simulink model "e_Aerodynamics_added"  (R2025b)
settings: Solver=ode23tb  StartTime=0.0  StopTime=20  MaxStep=0.001  RelTol=1e-3
model workspace (MAT data in the model file):
  init_r = 0
  init_vx = 0
  init_vy = 0
values from neighbouring files (symbols this model uses):
  Par =     [0_Load_data.mat]
  TireData =     [0_Load_data.mat]
libraries: simulink x3
(part 1 of 2)
settings Model: PauseTimes=0  PacingRate=0.001000  Creator=rajde  LastModifiedBy=vishal bhujbal
settings DataIOCC: SaveOutput=off  SaveTime=off
settings DebuggingCC: UnderSpecifiedDimensionMsg=warning

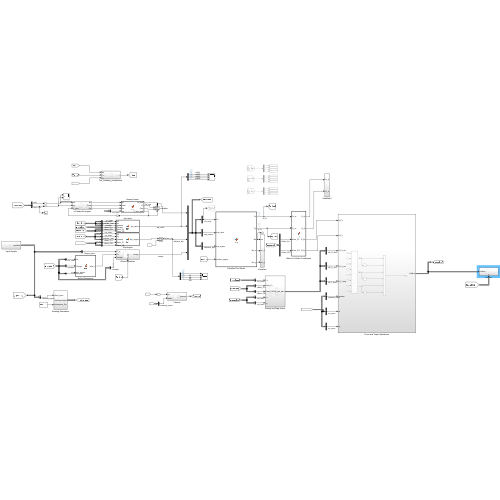
[thumbnail: Simulink's stored preview of the top-level diagram]
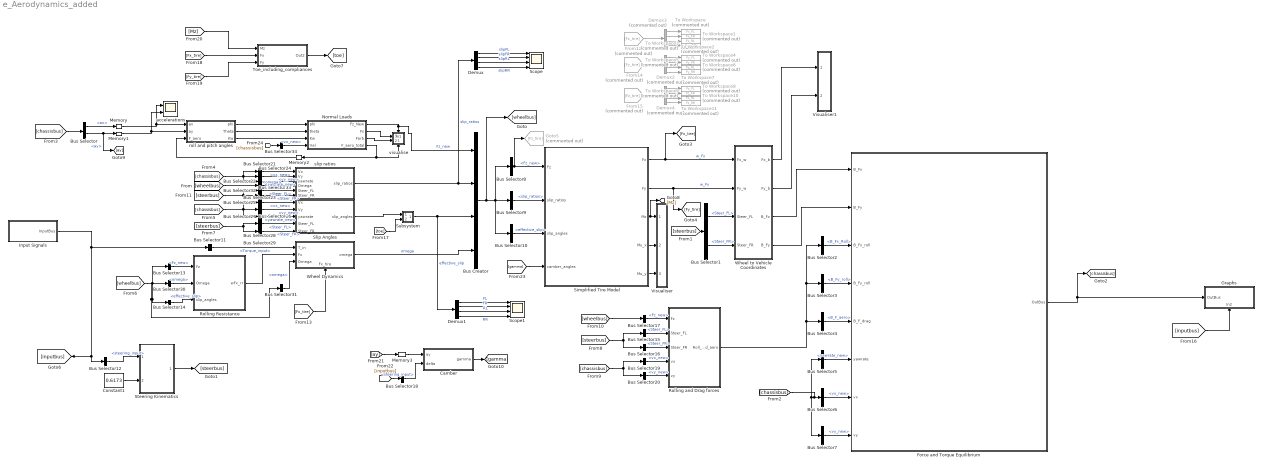
== system e_Aerodynamics_added ==
  Bus Creator : BusCreator  Inputs=4
  Bus Selector : BusSelector  OutputSignals=ax,ay
  Bus Selector1 : BusSelector  OutputSignals=Steer_FL,Steer_FR
  Bus Selector10 : BusSelector  OutputSignals=effective_slip
  Bus Selector11 : BusSelector  OutputSignals=Torque_input
  Bus Selector12 : BusSelector  OutputSignals=steering_input
  Bus Selector13 : BusSelector  OutputSignals=Fz_new
  Bus Selector14 : BusSelector  OutputSignals=effective_slip
  Bus Selector15 : BusSelector  OutputSignals=Steer_FL
  Bus Selector16 : BusSelector  OutputSignals=Steer_FR
  Bus Selector17 : BusSelector  OutputSignals=Fz_new
  Bus Selector18 : BusSelector  OutputSignals=steering_input
  Bus Selector{6,19,21,25,34} (5 alike) : BusSelector  OutputSignals=vx_new
  Bus Selector2 : BusSelector  OutputSignals=B_Fx_Roll
  Bus Selector{7,20,24,26} (4 alike) : BusSelector  OutputSignals=vy_new
  Bus Selector22 : BusSelector  OutputSignals=yawrate_new
  Bus Selector23 : BusSelector  OutputSignals=omega
  Bus Selector27 : BusSelector  OutputSignals=yawrate_new
  Bus Selector28 : BusSelector  OutputSignals=Steer_FL
  Bus Selector29 : BusSelector  OutputSignals=Steer_FR
  Bus Selector3 : BusSelector  OutputSignals=B_Fy_roll
  Bus Selector30 : BusSelector  OutputSignals=omega
  Bus Selector31 : BusSelector  OutputSignals=omega
  Bus Selector32 : BusSelector  OutputSignals=Steer_FL
  Bus Selector33 : BusSelector  OutputSignals=Steer_FR
  Bus Selector4 : BusSelector  OutputSignals=B_F_aero
  Bus Selector5 : BusSelector  OutputSignals=yawrate_new
  Bus Selector8 : BusSelector  OutputSignals=Fz_new
  Bus Selector9 : BusSelector  OutputSignals=slip_ratios
  Camber : Subsystem
  Constant1 : Constant  Value=0.6173
  Demux : Demux
  Demux1 : Demux
  Demux2 : Demux  Commented=on
  Demux3 : Demux  Commented=on
  Demux4 : Demux  Commented=on
  Force and Torque Equilibrium : Subsystem
  From12 : From  Commented=on  GotoTag=Fx_tire
  From14 : From  Commented=on  GotoTag=Fy_tire
  From15 : From  Commented=on  GotoTag=Fz_tire
  Goto5 : Goto  Commented=on  GotoTag=Fz_tire
  Graphs : Subsystem
      settings: PortSchema="{\"entries\":[{\"content\":{\"sides\":[{\"content\":{\"connectorIds\":[\"In1\"]},\"type\":\"ConnectorPlacement.EquallySpacedRectSide\",\"uuid\":\"0d7f1a6c-503e-4c9f-90e9-70f717dd7dfc\"},{\"content\":{\"side\":\"RIGHT\"},\"type\":\"ConnectorPlacement.EquallySpacedRectSide\",\"uuid\":\"62097468-b066-4e29-8f99-7427d14bee77\"},{\"content\":{\"side\":\"TOP\"},\"type\":\"ConnectorPlacement.EquallySpacedRectSide\",\"uuid\":\"2a3f381e-a201-4804-99b7-77b73504b102\"},{\"content\":{\"connectorIds\":[\"In2\"],\"side\":\"BOTTOM\"},\"type\":\"ConnectorPlacement.EquallySpacedRectSide\",\"uuid\":\"dae5de0a-879c-4844-a347-7056417d054f\"}]},\"type\":\"ConnectorPlacement.EquallySpacedConnector\",\"uuid\":\"aa2835d0-6748-4566-adf9-84e8214dd5a8\"}],\"packageUris\":[\"http://schema.mathworks.com/mf0/Connector/R2020b\"],\"version\":\"1.0\"}"
  Input Signals : Subsystem
  Memory : Memory  InheritSampleTime=on
  Memory1 : Memory  InheritSampleTime=on
  Memory2 : Memory  InheritSampleTime=on
  Memory3 : Memory
  Normal Loads : MATLAB Function  TreatAsAtomicUnit=on
  Rolling Resistance : MATLAB Function  TreatAsAtomicUnit=on
  Rolling and Drag forces : Subsystem
  Scope : Scope  NumInputPorts=4
      settings: ActiveDisplayYMinimum=-0.00902343797023162  ActiveDisplayYMaximum=0.049451714787091476  DataLoggingVariableName=ScopeData3
  Scope1 : Scope  NumInputPorts=4
      settings: ActiveDisplayYMinimum=-0.4830772017663526  ActiveDisplayYMaximum=0.53547210256097  DataLoggingVariableName=ScopeData4
  Simplified Tire Model : MATLAB Function  TreatAsAtomicUnit=on
  Slip Angles : MATLAB Function  TreatAsAtomicUnit=on
  Steering Kinematics : Subsystem
  Subsystem : Subsystem
  To Workspace : ToWorkspace  Commented=on  VariableName=Fx_FL  SaveFormat=Timeseries  SampleTime=-1
  To Workspace1 : ToWorkspace  Commented=on  VariableName=Fx_FR  SaveFormat=Timeseries  SampleTime=-1
  To Workspace10 : ToWorkspace  Commented=on  VariableName=Fz_RL  SaveFormat=Timeseries  SampleTime=-1
  To Workspace11 : ToWorkspace  Commented=on  VariableName=Fz_RR  SaveFormat=Timeseries  SampleTime=-1
  To Workspace2 : ToWorkspace  Commented=on  VariableName=Fx_RL  SaveFormat=Timeseries  SampleTime=-1
  To Workspace3 : ToWorkspace  Commented=on  VariableName=Fx_RR  SaveFormat=Timeseries  SampleTime=-1
  To Workspace4 : ToWorkspace  Commented=on  VariableName=Fy_FL  SaveFormat=Timeseries  SampleTime=-1
  To Workspace5 : ToWorkspace  Commented=on  VariableName=Fy_FR  SaveFormat=Timeseries  SampleTime=-1
  To Workspace6 : ToWorkspace  Commented=on  VariableName=Fy_RL  SaveFormat=Timeseries  SampleTime=-1
  To Workspace7 : ToWorkspace  Commented=on  VariableName=Fy_RR  SaveFormat=Timeseries  SampleTime=-1
  To Workspace8 : ToWorkspace  Commented=on  VariableName=Fz_FL  SaveFormat=Timeseries  SampleTime=-1
  To Workspace9 : ToWorkspace  Commented=on  VariableName=Fz_FR  SaveFormat=Timeseries  SampleTime=-1
  Toe_including_compliances : Subsystem
  Visualiser : Subsystem
  Visualiser1 : Subsystem
  Wheel Dynamics : Subsystem
      settings: PortSchema="{\"entries\":[{\"content\":{\"sides\":[{\"content\":{\"connectorIds\":[\"In1\",\"In2\",\"In3\"]},\"type\":\"ConnectorPlacement.EquallySpacedRectSide\",\"uuid\":\"f2e918e6-c6f6-4ec9-89f3-e2543a6374fd\"},{\"content\":{\"connectorIds\":[\"Out1\"],\"side\":\"RIGHT\"},\"type\":\"ConnectorPlacement.EquallySpacedRectSide\",\"uuid\":\"be700f5f-5cf3-4eec-a6f7-872bb7cd40f6\"},{\"content\":{\"side\":\"TOP\"},\"type\":\"ConnectorPlacement.EquallySpacedRectSide\",\"uuid\":\"c4f49273-9888-4d11-a98e-35dc6f585916\"},{\"content\":{\"connectorIds\":[\"In4\"],\"side\":\"BOTTOM\"},\"type\":\"ConnectorPlacement.EquallySpacedRectSide\",\"uuid\":\"8d2e7982-4362-4abb-b8fe-c155beeed1bc\"}]},\"type\":\"ConnectorPlacement.EquallySpacedConnector\",\"uuid\":\"4d6dafa1-905e-4e38-a48b-73a98e690073\"}],\"packageUris\":[\"http://schema.mathworks.com/mf0/Connector/R2020b\"],\"version\":\"1.0\"}"
  Wheel to Vehicle Coordinates : MATLAB Function  TreatAsAtomicUnit=on
  accelerations : Scope  NumInputPorts=2
      settings: ActiveDisplayYMinimum=-9.8753419220215122  ActiveDisplayYMaximum=20.918858613729107  DataLoggingVariableName=ScopeData12
  roll and pitch angles : Subsystem
  slip ratios : MATLAB Function  TreatAsAtomicUnit=on
  visualise : Subsystem
      settings: PortSchema="{\"entries\":[{\"content\":{\"sides\":[{\"content\":{\"connectorIds\":[\"In1\"]},\"type\":\"ConnectorPlacement.EquallySpacedRectSide\",\"uuid\":\"8366d134-d050-42cc-b256-e51a937b8428\"},{\"content\":{\"connectorIds\":[\"In4\"],\"side\":\"RIGHT\"},\"type\":\"ConnectorPlacement.EquallySpacedRectSide\",\"uuid\":\"98870c85-a760-468e-85de-3959de32b175\"},{\"content\":{\"connectorIds\":[\"In2\",\"In3\"],\"side\":\"TOP\"},\"type\":\"ConnectorPlacement.EquallySpacedRectSide\",\"uuid\":\"b49e1108-902f-401f-be37-4fefd9726c90\"}]},\"type\":\"ConnectorPlacement.EquallySpacedConnector\",\"uuid\":\"4200efe4-5812-4945-a73f-d6022d642a21\"}],\"packageUris\":[\"http://schema.mathworks.com/mf0/Connector/R2020b\"],\"version\":\"1.0\"}"
  wires:
  Simplified Tire Model/3(Mz) -> [Mz], Visualiser/1(mz)
  Simplified Tire Model/4(Mu_x) -> Visualiser/2(mu_x)
  Simplified Tire Model/5(Mu_y) -> Visualiser/3(mu_y)
  Simplified Tire Model/2(Fy) -> Wheel to Vehicle Coordinates/2(Fy_w), [Fy_tire]  "w_Fy"
  Simplified Tire Model/1(Fx) -> Wheel to Vehicle Coordinates/1(Fx_w), [Fx_tire]  "w_Fx"
  Wheel to Vehicle Coordinates/2(Fy_b) -> Visualiser1/2(Fy_b)
  Wheel to Vehicle Coordinates/1(Fx_b) -> Visualiser1/1(Fx_b)
  Wheel to Vehicle Coordinates/3(B_Fx) -> Force and Torque Equilibrium/1(B_Fx)
  Wheel to Vehicle Coordinates/4(B_Fy) -> Force and Torque Equilibrium/2(B_Fy)
  slip ratios/1(slip_ratios) -> Demux/1, Bus Creator/2  "slip_ratios"
  Wheel Dynamics/1(omega) -> Bus Creator/4  "omega"
  Bus Selector/1 -> Memory/1  "<ax>"
  Rolling Resistance/1(wFx_rr) -> Wheel Dynamics/2(Fx)
  Bus Selector1/1 -> Wheel to Vehicle Coordinates/3(Steer_FL)  "<Steer_FL>"
  Bus Selector1/2 -> Wheel to Vehicle Coordinates/4(Steer_FR)  "<Steer_FR>"
  Rolling and Drag forces/1(Roll_and_aero) -> Bus Selector2/1, Bus Selector3/1, Bus Selector4/1
  Bus Selector2/1 -> Force and Torque Equilibrium/3(B_Fx_roll)  "<B_Fx_Roll>"
  Bus Selector3/1 -> Force and Torque Equilibrium/4(B_Fy_roll)  "<B_Fy_roll>"
  Bus Selector4/1 -> Force and Torque Equilibrium/5(B_F_drag)  "<B_F_aero>"
  Bus Selector5/1 -> Force and Torque Equilibrium/6(yawrate)  "<yawrate_new>"
  Force and Torque Equilibrium/1(OutBus) -> [chassisbus], Graphs/1(OutBus)
  Bus Selector7/1 -> Force and Torque Equilibrium/8(vy)  "<vy_new>"
  Bus Selector6/1 -> Force and Torque Equilibrium/7(vx)  "<vx_new>"
  Bus Selector8/1 -> Goto5/1, Simplified Tire Model/1(Fz)  "<Fz_new>"
  Bus Selector10/1 -> Simplified Tire Model/3(slip_angles)  "<effective_slip>"
  Bus Selector9/1 -> Simplified Tire Model/2(slip_ratios)  "<slip_ratios>"
  Bus Creator/1 -> [wheelbus], Bus Selector10/1, Bus Selector8/1, Bus Selector9/1
  Bus Selector12/1 -> Steering Kinematics/1(Steer_Input)  "<steering_input>"
  Bus Selector11/1 -> Wheel Dynamics/1(T_in)  "<Torque_input>"
  Input Signals/1(InputBus) -> Bus Selector12/1, [inputbus], Bus Selector11/1
  Bus Selector14/1 -> Rolling Resistance/3(slip_angles)  "<effective_slip>"
  Bus Selector15/1 -> Rolling and Drag forces/2(Steer_FL)  "<Steer_FL>"
  Bus Selector16/1 -> Rolling and Drag forces/3(Steer_FR)  "<Steer_FR>"
  Constant1/1 -> Steering Kinematics/2(Ackermann_Pct)
  Bus Selector17/1 -> Rolling and Drag forces/1(Fz)  "<Fz_new>"
  Bus Selector19/1 -> Rolling and Drag forces/4(vx)  "<vx_new>"
  Bus Selector20/1 -> Rolling and Drag forces/5(vy)  "<vy_new>"
  Bus Selector21/1 -> slip ratios/1(Vx)  "<vx_new>"
  Bus Selector22/1 -> slip ratios/3(yawrate)  "<yawrate_new>"
  Bus Selector23/1 -> slip ratios/4(Omega)  "<omega>"
  Bus Selector25/1 -> Slip Angles/1(Vx)  "<vx_new>"
  Bus Selector26/1 -> Slip Angles/2(Vy)  "<vy_new>"
  Bus Selector27/1 -> Slip Angles/3(yawrate)  "<yawrate_new>"
  Bus Selector28/1 -> Slip Angles/4(Steer_FL)  "<Steer_FL>"
  Bus Selector29/1 -> Slip Angles/5(Steer_FR)  "<Steer_FR>"
  Steering Kinematics/1(Steering Angles) -> [steerbus]
  [steerbus] -> Bus Selector1/1
  [chassisbus] -> Bus Selector5/1, Bus Selector7/1, Bus Selector6/1
  [chassisbus] -> Bus Selector/1
  Bus Selector/2 -> Memory1/1, [ay]  "<ay>"
  [wheelbus] -> Bus Selector23/1
  [chassisbus] -> Bus Selector22/1, Bus Selector24/1, Bus Selector21/1
  [chassisbus] -> Bus Selector27/1, Bus Selector26/1, Bus Selector25/1
  [steerbus] -> Bus Selector29/1, Bus Selector28/1
  [wheelbus] -> Bus Selector13/1, Bus Selector30/1, Bus Selector14/1, Bus Selector31/1
  Bus Selector30/1 -> Rolling Resistance/2(Omega)  "<omega>"
  Bus Selector31/1 -> Wheel Dynamics/3(Omega)  "<omega>"
  [steerbus] -> Bus Selector16/1, Bus Selector15/1
  [chassisbus] -> Bus Selector20/1, Bus Selector19/1
  [wheelbus] -> Bus Selector17/1
  Demux/1 -> Scope/1  "slipFL"
  Demux/3 -> Scope/3  "slipRL"
  Demux/4 -> Scope/4  "slipRR"
  Demux/2 -> Scope/2  "slipFR"
  Demux1/1 -> Scope1/1  "FL"
  Demux1/2 -> Scope1/2  "FR"
  Demux1/4 -> Scope1/4  "RR"
  Demux1/3 -> Scope1/3  "RL"
  Bus Selector24/1 -> slip ratios/2(Vy)  "<vy_new>"
  Bus Selector33/1 -> slip ratios/6(Steer_FR)  "<Steer_FR>"
  [steerbus] -> Bus Selector32/1, Bus Selector33/1
  Bus Selector32/1 -> slip ratios/5(Steer_FL)  "<Steer_FL>"
  [Fx_tire] -> Wheel Dynamics/4(Fx_tire)
  Bus Selector13/1 -> Rolling Resistance/1(Fz)  "<Fz_new>"
  Demux2/2 -> To Workspace5/1
  Demux2/3 -> To Workspace6/1
  Demux3/3 -> To Workspace2/1
  Demux3/4 -> To Workspace3/1
  From12/1 -> Demux3/1
  From14/1 -> Demux2/1
  Demux3/2 -> To Workspace1/1
  Demux2/4 -> To Workspace7/1
  Demux3/1 -> To Workspace/1
  Demux2/1 -> To Workspace4/1
  Demux4/1 -> To Workspace8/1
  Demux4/4 -> To Workspace11/1
  Demux4/2 -> To Workspace9/1
  Demux4/3 -> To Workspace10/1
  From15/1 -> Demux4/1
  [inputbus] -> Graphs/2(In2)
  Slip Angles/1(slip_angles) -> Subsystem/1(slip_angles)
  [toe] -> Subsystem/2(toe)
  Subsystem/1(Out1) -> Demux1/1, Bus Creator/3  "effective_slip"
  [Mz] -> Toe_including_compliances/1(Mz)
  [Fx_tire] -> Toe_including_compliances/2(Fx)
  [Fy_tire] -> Toe_including_compliances/3(Fy)
  Toe_including_compliances/1(Out2) -> [toe]
  [ay] -> Memory3/1
  [inputbus] -> Bus Selector18/1
  Bus Selector18/1 -> Camber/2(delta)  "<steering_input>"
  Camber/1(gamma) -> [gamma]
  [gamma] -> Simplified Tire Model/4(camber_angles)
  roll and pitch angles/1(phi) -> Normal Loads/1(phi)
  roll and pitch angles/2(Theta) -> Normal Loads/2(theta)
  roll and pitch angles/3(Kw) -> Normal Loads/3(Kw)
  Normal Loads/1(Fz_New) -> Bus Creator/1, visualise/4(In1)  "Fz_new"
  Normal Loads/2(Fs) -> visualise/3(Fs)
  Normal Loads/3(Farb) -> visualise/2(Farb)
  Memory/1 -> accelerations/1, roll and pitch angles/1(ax)
  Memory1/1 -> roll and pitch angles/2(ay), accelerations/2
  Memory3/1 -> Camber/1(ay)
  Normal Loads/4(F_aero_total) -> visualise/1(F_aero_total), Memory2/1
  Memory2/1 -> roll and pitch angles/3(F_aero)
  [chassisbus] -> Bus Selector34/1
  Bus Selector34/1 -> Normal Loads/4(Vel)  "<vx_new>"

== system e_Aerodynamics_added/Camber ==
  ay : Inport
  delta : Inport  Port=2
  MATLAB Function : MATLAB Function  TreatAsAtomicUnit=on
  Mux : Mux
  gamma : Outport
  wires:
  MATLAB Function/1(gamma_FR) -> Mux/1
  MATLAB Function/2(gamma_FL) -> Mux/2
  MATLAB Function/3(gamma_RL) -> Mux/3
  MATLAB Function/4(gamma_RR) -> Mux/4
  Mux/1 -> gamma/1
  ay/1 -> MATLAB Function/1(ay)
  delta/1 -> MATLAB Function/2(delta)

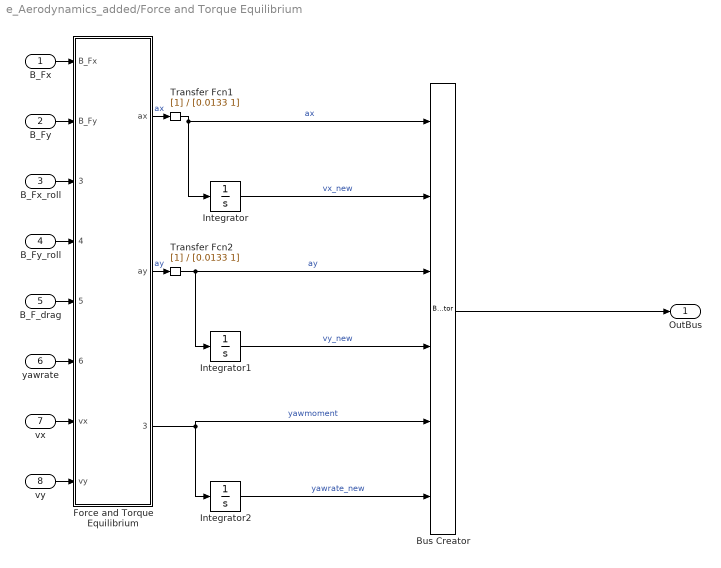
== system e_Aerodynamics_added/Force and Torque Equilibrium ==
  B_Fx : Inport
  B_Fy : Inport  Port=2
  B_Fx_roll : Inport  Port=3
  B_Fy_roll : Inport  Port=4
  B_F_drag : Inport  Port=5
  yawrate : Inport  Port=6
  vx : Inport  Port=7
  vy : Inport  Port=8
  Bus Creator : BusCreator  Inputs=6
  Force and Torque Equilibrium : MATLAB Function  TreatAsAtomicUnit=on
  Integrator : Integrator  LimitOutput=on  UpperSaturationLimit=1e6  LowerSaturationLimit=0
  Integrator1 : Integrator  LimitOutput=on  UpperSaturationLimit=1e6
  Integrator2 : Integrator  LimitOutput=on  UpperSaturationLimit=1e6
  Transfer Fcn1 : TransferFcn  Denominator=[0.0133 1]
  Transfer Fcn2 : TransferFcn  Denominator=[0.0133 1]
  OutBus : Outport
  wires:
  vy/1 -> Force and Torque Equilibrium/8(vy)
  B_Fx/1 -> Force and Torque Equilibrium/1(B_Fx)
  B_Fx_roll/1 -> Force and Torque Equilibrium/3(B_Fx_roll)
  B_F_drag/1 -> Force and Torque Equilibrium/5(B_F_drag)
  B_Fy/1 -> Force and Torque Equilibrium/2(B_Fy)
  B_Fy_roll/1 -> Force and Torque Equilibrium/4(B_Fy_roll)
  vx/1 -> Force and Torque Equilibrium/7(vx)
  Force and Torque Equilibrium/2(ay) -> Transfer Fcn2/1  "ay"
  Force and Torque Equilibrium/1(ax) -> Transfer Fcn1/1  "ax"
  Force and Torque Equilibrium/3(yawmoment) -> Integrator2/1, Bus Creator/5  "yawmoment"
  Integrator/1 -> Bus Creator/2  "vx_new"
  Integrator1/1 -> Bus Creator/4  "vy_new"
  Integrator2/1 -> Bus Creator/6  "yawrate_new"
  Bus Creator/1 -> OutBus/1
  yawrate/1 -> Force and Torque Equilibrium/6(yawrate)
  Transfer Fcn1/1 -> Integrator/1, Bus Creator/1  "ax"
  Transfer Fcn2/1 -> Integrator1/1, Bus Creator/3  "ay"

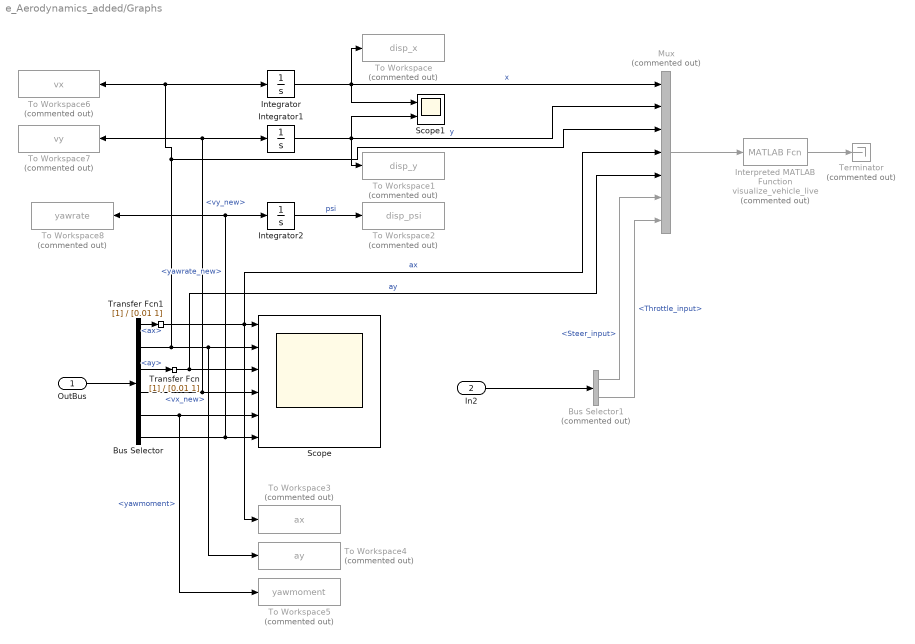
== system e_Aerodynamics_added/Graphs ==
  OutBus : Inport
  In2 : Inport  Port=2
  Bus Selector : BusSelector  OutputSignals=ax,vx_new,ay,vy_new,yawmoment,yawrate_new
  Bus Selector1 : BusSelector  Commented=on  OutputSignals=Steer_input,Throttle_input
  Integrator : Integrator
  Integrator1 : Integrator
  Integrator2 : Integrator
  Interpreted MATLAB Function : MATLABFcn  Commented=on  MATLABFcn=visualize_vehicle_live
  Mux : Mux  Commented=on  Inputs=7
  Scope : Scope  NumInputPorts=6
      settings: ActiveDisplayYMinimum=-1.8391798427639636  ActiveDisplayYMaximum=12.998606897592927  DataLoggingVariableName=ScopeData2
  Scope1 : Scope  NumInputPorts=2
      settings: ActiveDisplayYMinimum=-673.27901203322881  ActiveDisplayYMaximum=6059.5111082990607  DataLoggingVariableName=ScopeData7
  Terminator : Terminator  Commented=on
  To Workspace : ToWorkspace  Commented=on  VariableName=disp_x  SaveFormat=Timeseries  SampleTime=-1
  To Workspace1 : ToWorkspace  Commented=on  VariableName=disp_y  SaveFormat=Timeseries  SampleTime=-1
  To Workspace2 : ToWorkspace  Commented=on  VariableName=disp_psi  SaveFormat=Timeseries  SampleTime=-1
  To Workspace3 : ToWorkspace  Commented=on  VariableName=ax  SaveFormat=Timeseries  SampleTime=-1
  To Workspace4 : ToWorkspace  Commented=on  VariableName=ay  SaveFormat=Timeseries  SampleTime=-1
  To Workspace5 : ToWorkspace  Commented=on  VariableName=yawmoment  SaveFormat=Timeseries  SampleTime=-1
  To Workspace6 : ToWorkspace  Commented=on  VariableName=vx  SaveFormat=Timeseries  SampleTime=-1
  To Workspace7 : ToWorkspace  Commented=on  VariableName=vy  SaveFormat=Timeseries  SampleTime=-1
  To Workspace8 : ToWorkspace  Commented=on  VariableName=yawrate  SaveFormat=Timeseries  SampleTime=-1
  Transfer Fcn : TransferFcn  Denominator=[0.01 1]
  Transfer Fcn1 : TransferFcn  Denominator=[0.01 1]
  wires:
  OutBus/1 -> Bus Selector/1
  Bus Selector/1 -> Transfer Fcn1/1  "<ax>"
  Bus Selector/2 -> To Workspace6/1, Integrator/1, Mux/3, To Workspace4/1, Scope/2  "<vx_new>"
  Bus Selector/3 -> Transfer Fcn/1  "<ay>"
  Bus Selector/4 -> To Workspace7/1, Integrator1/1, Scope/4  "<vy_new>"
  Bus Selector/5 -> To Workspace5/1, Scope/5  "<yawmoment>"
  Bus Selector/6 -> To Workspace8/1, Integrator2/1, Scope/6  "<yawrate_new>"
  Integrator/1 -> Scope1/1, Mux/1, To Workspace/1  "x"
  Integrator1/1 -> Scope1/2, Mux/2, To Workspace1/1  "y"
  Integrator2/1 -> To Workspace2/1  "psi"
  Mux/1 -> Interpreted MATLAB Function/1
  Interpreted MATLAB Function/1 -> Terminator/1
  In2/1 -> Bus Selector1/1
  Bus Selector1/1 -> Mux/6  "<Steer_input>"
  Bus Selector1/2 -> Mux/7  "<Throttle_input>"
  Transfer Fcn/1 -> Mux/5, Scope/3  "ay"
  Transfer Fcn1/1 -> To Workspace3/1, Scope/1, Mux/4  "ax"

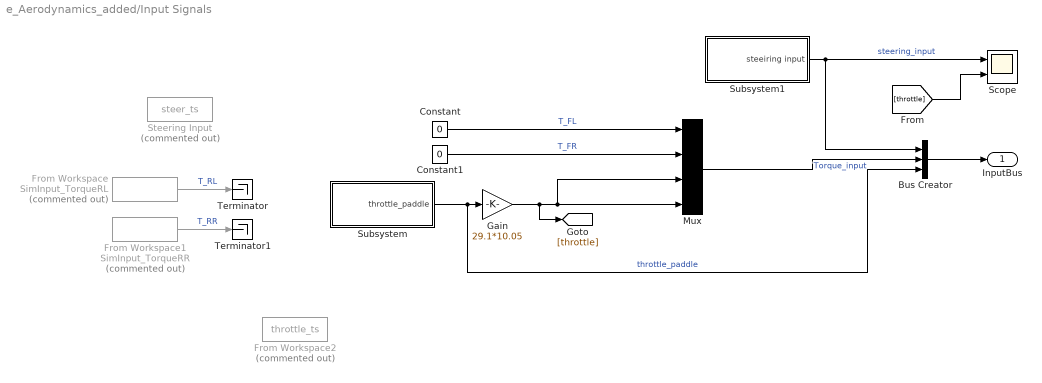
== system e_Aerodynamics_added/Input Signals ==
  Bus Creator : BusCreator  Inputs=3
  Constant : Constant  Value=0
  Constant1 : Constant  Value=0
  From Workspace : FromWorkspace  Commented=on  VariableName=SimInput_TorqueRL
  From Workspace1 : FromWorkspace  Commented=on  VariableName=SimInput_TorqueRR
  From Workspace2 : FromWorkspace  Commented=on  VariableName=throttle_ts
  Gain : Gain  Gain=29.1*10.05
  Mux : Mux
  Scope : Scope  NumInputPorts=2
      settings: ActiveDisplayYMinimum=-0.054541539124822784  ActiveDisplayYMaximum=0.49087385212340517  DataLoggingVariableName=ScopeData8
  Steering Input : FromWorkspace  Commented=on  VariableName=steer_ts
  Subsystem : Subsystem
  Subsystem1 : Subsystem
  Terminator : Terminator
  Terminator1 : Terminator
  InputBus : Outport
  wires:
  Bus Creator/1 -> InputBus/1
  Constant/1 -> Mux/1  "T_FL"
  Constant1/1 -> Mux/2  "T_FR"
  Mux/1 -> Bus Creator/2  "Torque_input"
  From Workspace1/1 -> Terminator1/1  "T_RR"
  From Workspace/1 -> Terminator/1  "T_RL"
  Gain/1 -> [throttle], Mux/4, Mux/3
  [throttle] -> Scope/2
  Subsystem/1(throttle_paddle) -> Bus Creator/3, Gain/1  "throttle_paddle"
  Subsystem1/1(steeiring input) -> Bus Creator/1, Scope/1  "steering_input"

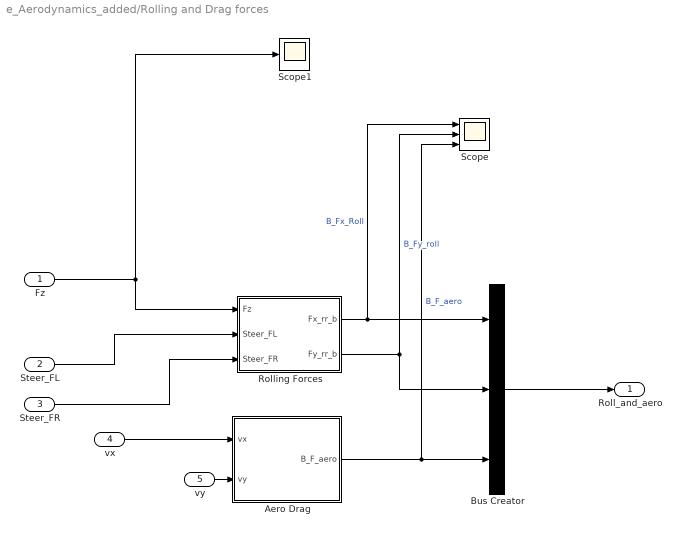
== system e_Aerodynamics_added/Rolling and Drag forces ==
  Fz : Inport
  Steer_FL : Inport  Port=2
  Steer_FR : Inport  Port=3
  vx : Inport  Port=4
  vy : Inport  Port=5
  Aero Drag : MATLAB Function  TreatAsAtomicUnit=on
  Bus Creator : BusCreator  Inputs=3
  Rolling Forces : MATLAB Function  TreatAsAtomicUnit=on
  Scope : Scope  NumInputPorts=3
      settings: ActiveDisplayYMinimum=-84.954759082659436  ActiveDisplayYMaximum=8.7114722532307756  DataLoggingVariableName=ScopeData5
  Scope1 : Scope
      settings: ActiveDisplayYMinimum=-1  ActiveDisplayYMaximum=1  DataLoggingVariableName=ScopeData6
  Roll_and_aero : Outport
  wires:
  Steer_FL/1 -> Rolling Forces/2(Steer_FL)
  vx/1 -> Aero Drag/1(vx)
  Fz/1 -> Scope1/1, Rolling Forces/1(Fz)
  Aero Drag/1(B_F_aero) -> Bus Creator/3, Scope/3  "B_F_aero"
  Rolling Forces/1(Fx_rr_b) -> Scope/1, Bus Creator/1  "B_Fx_Roll"
  Steer_FR/1 -> Rolling Forces/3(Steer_FR)
  vy/1 -> Aero Drag/2(vy)
  Rolling Forces/2(Fy_rr_b) -> Bus Creator/2, Scope/2  "B_Fy_roll"
  Bus Creator/1 -> Roll_and_aero/1

== system e_Aerodynamics_added/Steering Kinematics ==
  Steer_Input : Inport
  Ackermann_Pct : Inport  Port=2
  Bus Creator1 : BusCreator  Inputs=2
  Steering Kinematics : MATLAB Function  TreatAsAtomicUnit=on
  Steering Angles : Outport
  wires:
  Steering Kinematics/1(Steer_FL) -> Bus Creator1/1  "Steer_FL"
  Steer_Input/1 -> Steering Kinematics/1(Steer_Input)
  Steering Kinematics/2(Steer_FR) -> Bus Creator1/2  "Steer_FR"
  Ackermann_Pct/1 -> Steering Kinematics/2(Ackermann_Pct)
  Bus Creator1/1 -> Steering Angles/1

== system e_Aerodynamics_added/Subsystem ==
  slip_angles : Inport
  toe : Inport  Port=2
  Subtract : Sum  Inputs=+-
  Out1 : Outport
  wires:
  slip_angles/1 -> Subtract/1
  toe/1 -> Subtract/2
  Subtract/1 -> Out1/1

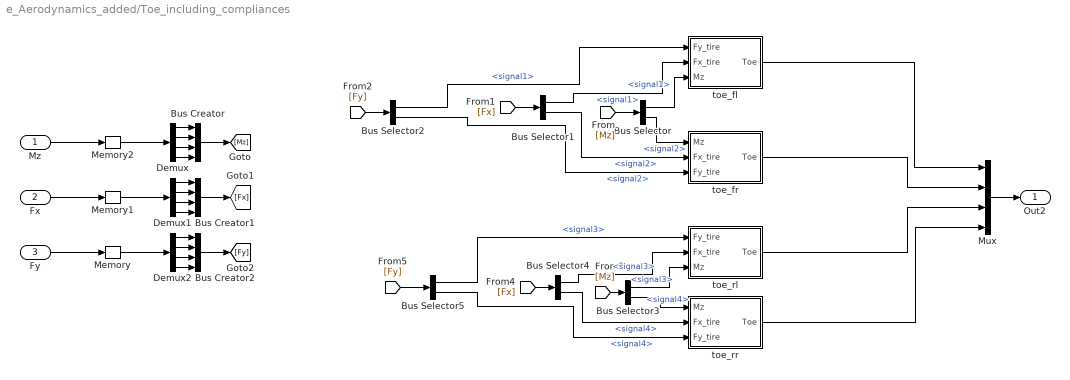
== system e_Aerodynamics_added/Toe_including_compliances ==
  Mz : Inport
  Fx : Inport  Port=2
  Fy : Inport  Port=3
  Bus Creator : BusCreator  Inputs=4
  Bus Creator1 : BusCreator  Inputs=4
  Bus Creator2 : BusCreator  Inputs=4
  Bus Selector : BusSelector  OutputSignals=signal1,signal2
  Bus Selector1 : BusSelector  OutputSignals=signal1,signal2
  Bus Selector2 : BusSelector  OutputSignals=signal1,signal2
  Bus Selector3 : BusSelector  OutputSignals=signal3,signal4
  Bus Selector4 : BusSelector  OutputSignals=signal3,signal4
  Bus Selector5 : BusSelector  OutputSignals=signal3,signal4
  Demux : Demux
  Demux1 : Demux
  Demux2 : Demux
  Memory : Memory
  Memory1 : Memory
  Memory2 : Memory
  Mux : Mux
  toe_fl : MATLAB Function  TreatAsAtomicUnit=on
  toe_fr : MATLAB Function  TreatAsAtomicUnit=on
  toe_rl : MATLAB Function  TreatAsAtomicUnit=on
  toe_rr : MATLAB Function  TreatAsAtomicUnit=on
  Out2 : Outport
  wires:
  Mz/1 -> Memory2/1
  Demux/1 -> Bus Creator/1
  Demux/2 -> Bus Creator/2
  Demux/3 -> Bus Creator/3
  Demux/4 -> Bus Creator/4
  Bus Creator/1 -> [Mz]
  [Mz] -> Bus Selector/1
  Bus Selector/1 -> toe_fl/3(Mz)  "<signal1>"
  Bus Selector/2 -> toe_fr/1(Mz)  "<signal2>"
  Fx/1 -> Memory1/1
  Demux1/1 -> Bus Creator1/1
  Demux1/2 -> Bus Creator1/2
  Demux1/3 -> Bus Creator1/3
  Demux1/4 -> Bus Creator1/4
  Bus Creator1/1 -> [Fx]
  Fy/1 -> Memory/1
  Demux2/1 -> Bus Creator2/1
  Demux2/2 -> Bus Creator2/2
  Demux2/3 -> Bus Creator2/3
  Demux2/4 -> Bus Creator2/4
  Bus Creator2/1 -> [Fy]
  [Fx] -> Bus Selector1/1
  Bus Selector1/1 -> toe_fl/2(Fx_tire)  "<signal1>"
  Bus Selector1/2 -> toe_fr/2(Fx_tire)  "<signal2>"
  [Fy] -> Bus Selector2/1
  Bus Selector2/1 -> toe_fl/1(Fy_tire)  "<signal1>"
  Bus Selector2/2 -> toe_fr/3(Fy_tire)  "<signal2>"
  Bus Selector3/1 -> toe_rl/3(Mz)  "<signal3>"
  [Mz] -> Bus Selector3/1
  [Fx] -> Bus Selector4/1
  [Fy] -> Bus Selector5/1
  Bus Selector3/2 -> toe_rr/1(Mz)  "<signal4>"
  Bus Selector4/1 -> toe_rl/2(Fx_tire)  "<signal3>"
  Bus Selector4/2 -> toe_rr/2(Fx_tire)  "<signal4>"
  Bus Selector5/1 -> toe_rl/1(Fy_tire)  "<signal3>"
  Bus Selector5/2 -> toe_rr/3(Fy_tire)  "<signal4>"
  toe_fl/1(Toe) -> Mux/1
  toe_fr/1(Toe) -> Mux/2
  toe_rl/1(Toe) -> Mux/3
  toe_rr/1(Toe) -> Mux/4
  Mux/1 -> Out2/1
  Memory/1 -> Demux2/1
  Memory1/1 -> Demux1/1
  Memory2/1 -> Demux/1

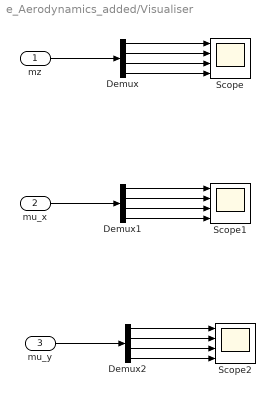
== system e_Aerodynamics_added/Visualiser ==
  mz : Inport
  mu_x : Inport  Port=2
  mu_y : Inport  Port=3
  Demux : Demux
  Demux1 : Demux
  Demux2 : Demux
  Scope : Scope  NumInputPorts=4
      settings: ActiveDisplayYMinimum=-1  ActiveDisplayYMaximum=1
  Scope1 : Scope  NumInputPorts=4
  Scope2 : Scope  NumInputPorts=4
  wires:
  mz/1 -> Demux/1
  Demux/1 -> Scope/1
  Demux/2 -> Scope/2
  Demux/3 -> Scope/3
  Demux/4 -> Scope/4
  Demux1/3 -> Scope1/3
  Demux1/2 -> Scope1/2
  mu_x/1 -> Demux1/1
  Demux1/1 -> Scope1/1
  Demux1/4 -> Scope1/4
  Demux2/3 -> Scope2/3
  Demux2/2 -> Scope2/2
  mu_y/1 -> Demux2/1
  Demux2/1 -> Scope2/1
  Demux2/4 -> Scope2/4

== system e_Aerodynamics_added/Visualiser1 ==
  Fx_b : Inport
  Fy_b : Inport  Port=2
  Demux : Demux
  Demux1 : Demux
  Scope : Scope  NumInputPorts=4
      settings: ActiveDisplayYMinimum=-1417.5016884545366  ActiveDisplayYMaximum=759.32056463381321
  Scope1 : Scope  NumInputPorts=4
      settings: ActiveDisplayYMinimum=-1  ActiveDisplayYMaximum=1
  wires:
  Fx_b/1 -> Demux/1
  Demux/1 -> Scope/1  "Fx_fl"
  Demux/2 -> Scope/2  "Fx_fr"
  Demux/3 -> Scope/3  "Fx_rl"
  Demux/4 -> Scope/4  "Fx_rr"
  Demux1/3 -> Scope1/3
  Demux1/2 -> Scope1/2
  Fy_b/1 -> Demux1/1
  Demux1/1 -> Scope1/1
  Demux1/4 -> Scope1/4

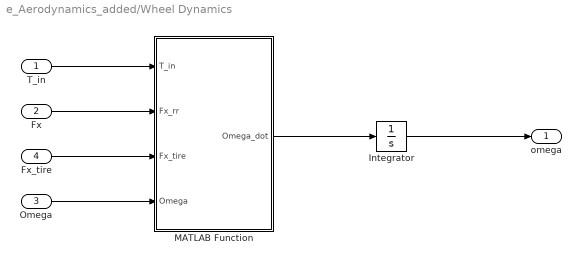
== system e_Aerodynamics_added/Wheel Dynamics ==
  T_in : Inport
  Fx : Inport  Port=2
  Omega : Inport  Port=3
  Fx_tire : Inport  Port=4
  Integrator : Integrator  LimitOutput=on  UpperSaturationLimit=1e6
  MATLAB Function : MATLAB Function  TreatAsAtomicUnit=on
  omega : Outport
  wires:
  Integrator/1 -> omega/1
  T_in/1 -> MATLAB Function/1(T_in)
  Fx/1 -> MATLAB Function/2(Fx_rr)
  Omega/1 -> MATLAB Function/4(Omega)
  MATLAB Function/1(Omega_dot) -> Integrator/1
  Fx_tire/1 -> MATLAB Function/3(Fx_tire)

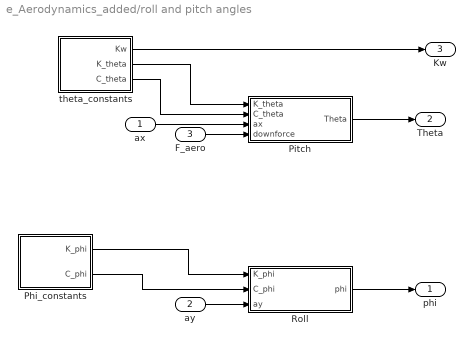
== system e_Aerodynamics_added/roll and pitch angles ==
  ax : Inport
  ay : Inport  Port=2
  F_aero : Inport  Port=3
  Phi_constants : MATLAB Function  TreatAsAtomicUnit=on
  Pitch : Subsystem
  Roll : Subsystem
  theta_constants : MATLAB Function  TreatAsAtomicUnit=on
  phi : Outport
  Theta : Outport  Port=2
  Kw : Outport  Port=3
  wires:
  ax/1 -> Pitch/3(ax)
  Phi_constants/1(K_phi) -> Roll/1(K_phi)
  Phi_constants/2(C_phi) -> Roll/2(C_phi)
  ay/1 -> Roll/3(ay)
  Roll/1(phi) -> phi/1
  Pitch/1(Theta) -> Theta/1
  theta_constants/1(Kw) -> Kw/1
  theta_constants/2(K_theta) -> Pitch/1(K_theta)
  theta_constants/3(C_theta) -> Pitch/2(C_theta)
  F_aero/1 -> Pitch/4(downforce)

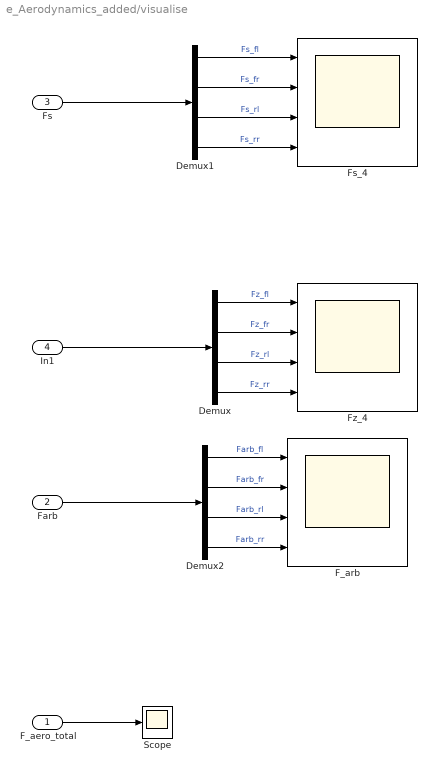
== system e_Aerodynamics_added/visualise ==
  F_aero_total : Inport
  Farb : Inport  Port=2
  Fs : Inport  Port=3
  In1 : Inport  Port=4
  Demux : Demux
  Demux1 : Demux
  Demux2 : Demux
  F_arb : Scope  NumInputPorts=4
      settings: ActiveDisplayYMinimum=-157.42008690270848  ActiveDisplayYMaximum=71.736384315929655  DataLoggingVariableName=ScopeData9
  Fs_4 : Scope  NumInputPorts=4
      settings: ActiveDisplayYMinimum=-337.10158174249347  ActiveDisplayYMaximum=241.329196269166  DataLoggingVariableName=ScopeData11
  Fz_4 : Scope  NumInputPorts=4
      settings: ActiveDisplayYMinimum=512.60798070216572  ActiveDisplayYMaximum=1526.8590967988266  DataLoggingVariableName=ScopeData10
  Scope : Scope
      settings: ActiveDisplayYMinimum=-184.57086138075974  ActiveDisplayYMaximum=1661.1377524268378  DataLoggingVariableName=ScopeData13
  wires:
  In1/1 -> Demux/1
  Demux/1 -> Fz_4/1  "Fz_fl"
  Demux/2 -> Fz_4/2  "Fz_fr"
  Demux/3 -> Fz_4/3  "Fz_rl"
  Demux/4 -> Fz_4/4  "Fz_rr"
  Demux1/1 -> Fs_4/1  "Fs_fl"
  Demux1/2 -> Fs_4/2  "Fs_fr"
  Demux1/3 -> Fs_4/3  "Fs_rl"
  Demux1/4 -> Fs_4/4  "Fs_rr"
  Demux2/1 -> F_arb/1  "Farb_fl"
  Demux2/2 -> F_arb/2  "Farb_fr"
  Demux2/3 -> F_arb/3  "Farb_rl"
  Demux2/4 -> F_arb/4  "Farb_rr"
  Farb/1 -> Demux2/1
  Fs/1 -> Demux1/1
  F_aero_total/1 -> Scope/1

== system e_Aerodynamics_added/Input Signals/Subsystem ==
  Ramp : simulink/Sources/Ramp  slope=1/6  start=0  InitialOutput=0
  Saturation : Saturate  UpperLimit=1  LowerLimit=0
  throttle_paddle : Outport
  wires:
  Ramp/1 -> Saturation/1
  Saturation/1 -> throttle_paddle/1

== system e_Aerodynamics_added/Input Signals/Subsystem1 ==
  Clock : Clock
  Ramp : simulink/Sources/Ramp  slope=-pi/30  start=10  InitialOutput=pi/6
  Ramp1 : simulink/Sources/Ramp  slope=pi/30  start=5  InitialOutput=0
  Saturation : Saturate  UpperLimit=25*pi/180  LowerLimit=0
  Switch : Switch  Criteria=u2 > Threshold  Threshold=10  SaturateOnIntegerOverflow=off  InputSameDT=off
  steeiring input : Outport
  wires:
  Ramp1/1 -> Switch/3
  Clock/1 -> Switch/2
  Ramp/1 -> Switch/1
  Switch/1 -> Saturation/1
  Saturation/1 -> steeiring input/1

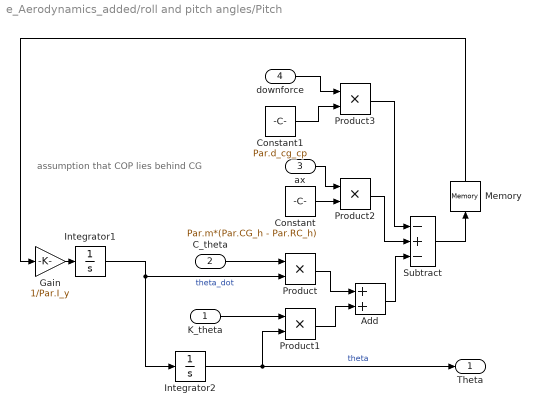
== system e_Aerodynamics_added/roll and pitch angles/Pitch ==
  note: assumption that COP lies behind CG
  K_theta : Inport
  C_theta : Inport  Port=2
  ax : Inport  Port=3
  downforce : Inport  Port=4
  Add : Sum
  Constant : Constant  Value=Par.m*(Par.CG_h - Par.RC_h)
  Constant1 : Constant  Value=Par.d_cg_cp
  Gain : Gain  Gain=1/Par.I_y
  Integrator1 : Integrator
  Integrator2 : Integrator
  Memory : Memory
  Product{,1..3} (4 alike) : Product
  Subtract : Sum  Inputs=-+-
  Theta : Outport
  wires:
  Gain/1 -> Integrator1/1
  Integrator1/1 -> Product/2, Integrator2/1  "theta_dot"
  C_theta/1 -> Product/1
  Integrator2/1 -> Theta/1, Product1/2  "theta"
  K_theta/1 -> Product1/1
  Product/1 -> Add/1
  Product1/1 -> Add/2
  ax/1 -> Product2/1
  Constant/1 -> Product2/2
  Product2/1 -> Subtract/2
  Add/1 -> Subtract/3
  Subtract/1 -> Memory/1
  Memory/1 -> Gain/1
  downforce/1 -> Product3/1
  Constant1/1 -> Product3/2
  Product3/1 -> Subtract/1

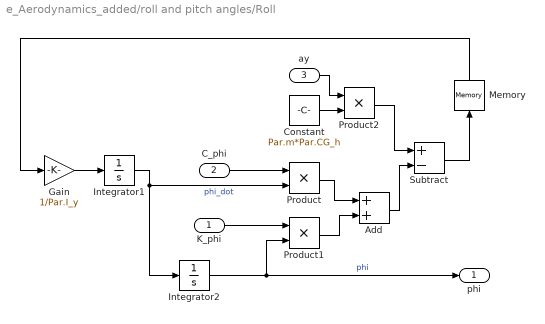
== system e_Aerodynamics_added/roll and pitch angles/Roll ==
  K_phi : Inport
  C_phi : Inport  Port=2
  ay : Inport  Port=3
  Add : Sum
  Constant : Constant  Value=Par.m*Par.CG_h
  Gain : Gain  Gain=1/Par.I_y
  Integrator1 : Integrator
  Integrator2 : Integrator
  Memory : Memory
  Product : Product
  Product1 : Product
  Product2 : Product
  Subtract : Sum  Inputs=+-
  phi : Outport
  wires:
  Subtract/1 -> Memory/1
  Add/1 -> Subtract/2
  Product2/1 -> Subtract/1
  Constant/1 -> Product2/2
  ay/1 -> Product2/1
  Product1/1 -> Add/2
  Product/1 -> Add/1
  K_phi/1 -> Product1/1
  Integrator2/1 -> Product1/2, phi/1  "phi"
  C_phi/1 -> Product/1
  Integrator1/1 -> Integrator2/1, Product/2  "phi_dot"
  Gain/1 -> Integrator1/1
  Memory/1 -> Gain/1

== matlab function e_Aerodynamics_added/Wheel Dynamics/MATLAB Function ==
  data: T_in input; Omega_dot output; Fx_rr input; Fx_tire input; Omega input; Par parameter
function Omega_dot = fcn(T_in, Fx_rr,Fx_tire, Omega, Par)
%#codegen

    % 1. Constants
    R = Par.R0;
    Iw = Par.I_wheel;

    % 2. Separate Drive and Brake components

    T_drive = max(T_in, 0); 
    
    % T_brake is the magnitude of the negative part of T_in
    T_brake_mag = abs(min(T_in, 0));
    

    Rotation_Dir = tanh(10 * Omega);

    % 4. Calculate Net Torque
    T_tire_reaction = abs(Fx_rr .* R);
    T_tire = Fx_tire .*R;
    T_damping = 0.1*Omega;
    T_net = T_drive - (T_brake_mag .* Rotation_Dir) - (T_tire_reaction.*Rotation_Dir) -T_tire - T_damping;

    % 5. Compute Angular Acceleration
    Omega_dot = T_net ./ Iw;

end

== matlab function e_Aerodynamics_added/Rolling Resistance ==
  data: Fz input; wFx_rr output; Omega input; slip_angles input; Par parameter
function wFx_rr  = fcn(Fz, Omega,slip_angles, Par)
%#codegen

    % 1. Calculate Total Magnitude
    F_mag = Par.C_rr .* abs(Fz);

    % 2. Determine Direction
    Dir = tanh(10 * Omega);

    
    % X-Component: Resists Spin (Torque generating)
    % wFx = -Magnitude * Direction * cos(Alpha)
    wFx_rr = -F_mag .*Dir.* cos(slip_angles);

end

== matlab function e_Aerodynamics_added/Rolling and Drag forces/Rolling Forces ==
  data: Fz input; Fx_rr_b output; Steer_FL input; Steer_FR input; Fy_rr_b output; Par parameter
function [Fx_rr_b, Fy_rr_b] = fcn(Fz, Steer_FL, Steer_FR, Par)

    %#codegen

    % 1. Setup
    C_rr = Par.C_rr; 
    
    % Construct Steering Vector (Assuming Rear Steer = 0)
    Delta = [Steer_FL; Steer_FR; 0; 0];

    % Initialize Outputs
    Fx_rr_b = zeros(4, 1);
    Fy_rr_b = zeros(4, 1);

    % 2. Calculate & Resolve Forces (Vectorized Loop)
    for i = 1:4
        
        % Magnitude (Always positive Fz)
        F_mag = C_rr * abs(Fz(i));
        
        % B. Define Force Vector in Wheel Frame
        F_xw = -F_mag;
        F_yw = 0;
        
        % C. Transform to Body Frame (Rotation)
        d = Delta(i);
        c = cos(d);
        s = sin(d);
        
        % Rotate: F_body = Rz(delta) * F_wheel
        % Fx_b = Fx_w*cos - Fy_w*sin
        Fx_rr_b(i) = F_xw * c - F_yw * s;
        
        % Fy_b = Fx_w*sin + Fy_w*cos
        Fy_rr_b(i) = F_xw * s + F_yw * c;
    end

end

== matlab function e_Aerodynamics_added/Force and Torque Equilibrium/Force and Torque Equilibrium ==
  data: B_Fx input; ax output size=1; ay output size=1; B_Fy input; B_Fx_roll input; B_Fy_roll input; B_F_drag input; yawrate input; vx input; vy input; yawmoment output size=1; Par parameter
function [ax, ay, yawmoment] = fcn(B_Fx, B_Fy, B_Fx_roll, B_Fy_roll, B_F_drag, yawrate, vx, vy, Par)
%#codegen

    % 1. Geometry Setup
    m = Par.m;
    Iz = Par.Iz;
    a = Par.a;     % CG to Front Axle
    b = Par.b;     % CG to Rear Axle
    half_T = Par.TW / 2; 

    % 2. Combine Forces at Each Corner (Traction + Rolling)

    Fx_total = B_Fx + B_Fx_roll; 
    Fy_total = B_Fy + B_Fy_roll; 
    
    % 3. Force Equilibrium
    Sigma_Fx = sum(Fx_total) - B_F_drag(1);
    Sigma_Fy = sum(Fy_total) ;
    
    % 4. Linear Accelerations 

    ax = (Sigma_Fx / m) + (vy * yawrate);
    ay = (Sigma_Fy / m) - (vx * yawrate);
    
    % --- Front Left (Index 1) ---
    % x = +a, y = +half_T
    M_FL = (a * Fy_total(1)) - (half_T * Fx_total(1));
    
    % --- Front Right (Index 2) ---
    % x = +a, y = -half_T
    % Note: -(-half_T) becomes +half_T
    M_FR = (a * Fy_total(2)) - (-half_T * Fx_total(2));
    
    % --- Rear Left (Index 3) ---
    % x = -b, y = +half_T
    M_RL = (-b * Fy_total(3)) - (half_T * Fx_total(3));
    
    % --- Rear Right (Index 4) ---
    % x = -b, y = -half_T
    M_RR = (-b * Fy_total(4)) - (-half_T * Fx_total(4));
    
    % 6. Total Yaw Moment & Acceleration
    Sigma_Mz = M_FL + M_FR + M_RL + M_RR;
    yawmoment = Sigma_Mz / Iz;

end

== matlab function e_Aerodynamics_added/Rolling and Drag forces/Aero Drag ==
  data: vx input; B_F_aero output; vy input; Par parameter
function B_F_aero = fcn(vx, vy, Par)

    %#codegen
    % AERODYNAMIC DRAG (Body Frame)
    % Calculates drag vector acting on the CG.
%
% Inputs:
%   vx, vy : Vehicle Velocities in Body Frame [m/s]
%   Par    : Parameters (.Cd, .Area, .rho, .C_side)
%
% Output:
%   B_F_aero : [Fx; Fy; 0] Aerodynamic Force Vector [N]

    % 1. Longitudinal Drag (Standard)
    % Fx = -0.5 * rho * Cd * Area * vx^2
    % Usage: sign(vx) ensures drag always opposes motion
    Fx_drag = 0.5 * Par.rho * Par.Cd * Par.Area * vx * abs(vx);

    % 2. Lateral Drag (Side Force) - Optional
    % Only relevant if sliding significantly.
    % If Par.C_side is not defined, calculate as 0.
    if isfield(Par, 'C_side') && Par.C_side > 0
        % Side area is often approx same as Frontal Area or larger
        % Fy = -0.5 * rho * C_side * Area_Side * vy^2
        Fy_drag = -0.5 * Par.rho * Par.C_side * Par.Area * vy * abs(vy);
    else
        Fy_drag = 0;
    end
    
    % 3. Output Vector for Equilibrium Block
    B_F_aero = [Fx_drag; Fy_drag; 0];

end

== matlab function e_Aerodynamics_added/Toe_including_compliances/toe_fl ==
  data: Fy_tire input; Fx_tire input; Toe output; Mz input; Par parameter
function Toe = fcn(Fy_tire,Fx_tire,Mz,Par)

Toe= Par.Toe_F_static + Par.C_fx_toe.*Fx_tire + Par.C_Fy_toe.*Fy_tire + Par.C_Mz_toe.*Mz;

== matlab function e_Aerodynamics_added/Toe_including_compliances/toe_fr ==
  data: Toe output; Mz input; Fx_tire input; Fy_tire input; Par parameter
function Toe = fcn(Mz,Fx_tire,Fy_tire,Par)

Toe= Par.Toe_F_static + Par.C_fx_toe.*Fx_tire + Par.C_Fy_toe.*Fy_tire + Par.C_Mz_toe.*Mz;

== matlab function e_Aerodynamics_added/Toe_including_compliances/toe_rl ==
  data: Fy_tire input; Fx_tire input; Toe output; Mz input; Par parameter
function Toe = fcn(Fy_tire,Fx_tire,Mz,Par)

Toe = Par.Toe_R_static + Par.C_fx_toe.*Fx_tire + Par.C_Fy_toe.*Fy_tire + Par.C_Mz_toe.*Mz;

== matlab function e_Aerodynamics_added/Toe_including_compliances/toe_rr ==
  data: Toe output; Mz input; Fx_tire input; Fy_tire input; Par parameter
function Toe = fcn(Mz,Fx_tire,Fy_tire,Par)

Toe = Par.Toe_R_static + Par.C_fx_toe.*Fx_tire + Par.C_Fy_toe.*Fy_tire + Par.C_Mz_toe.*Mz;

== matlab function e_Aerodynamics_added/Camber/MATLAB Function ==
  data: gamma_FR output; ay input; gamma_FL output; gamma_RL output; gamma_RR output; delta input; Par parameter
function [gamma_FR,gamma_FL,gamma_RL,gamma_RR] = fcn(ay,delta,Par)
par = Par;

%% Static camber
gamma_static = par.Camber_static;
% track_width = par.TW;
%% SUSPENSION ROLL STIFFNESS
k_phi1 = 10014;  % front axle roll stiffness (Nm/rad)
k_phi2 = 11466;  % rear axle roll stiffness (Nm/rad)

%% ROLL CENTER HEIGHTS
q1 = 0.062;      % front roll center height (m)
q2 = 0.091;      % rear roll center height (m)

%% CAMBER GEOMETRY
b1 = 0.20;       % front IC horizontal distance (m)
b2 = 0.22;       % rear IC horizontal distance (m)

%% TOTAL ROLL STIFFNESS
k_phi_total = k_phi1 + k_phi2;

%% TOTAL VEHICLE ROLL ANGLE
phi = par.m.*ay.*par.CG_h / k_phi_total;   % rad

%% AXLE ROLL ANGLES
phi_s1 = phi * (k_phi1 / k_phi_total);   % front suspension roll
phi_s2 = phi * (k_phi2 / k_phi_total);   % rear suspension roll

% Zwc_f = track_width.*0.5.*phi_s1;
% Zwc_r = track_width.*0.5.*phi_s2;
%% CAMBER GAIN COEFFICIENTS
k_gamma_f = - (q1 - b1) / b1;   % front
k_gamma_r = - (q2 - b2) / b2;   % rear

%% Camber due to roll on front axle
delta_gamma_roll_f = k_gamma_f * phi_s1;

%% Camber due to roll on rear axle
delta_gamma_roll_r = k_gamma_r * phi_s2;

%% Camber gain due to heave
% delta_gamma_heave_f = atan(Zwc_f/par.L_fvsa);
% delta_gamma_heave_r = atan(Zwc_r/par.L_fvsa);

%% Camber due to caster 
delta_gamma_caster = atan(tan(par.Caster_static).*sin(delta));

%% Camber angle
gamma_FL = gamma_static + delta_gamma_roll_f + delta_gamma_caster;
gamma_FR = gamma_static - (delta_gamma_roll_f + delta_gamma_caster);
gamma_RL = gamma_static + delta_gamma_roll_r + delta_gamma_caster;
gamma_RR = gamma_static - (delta_gamma_roll_r + delta_gamma_caster);

== matlab function e_Aerodynamics_added/roll and pitch angles/theta_constants ==
  data: Kw output; K_theta output; C_theta output; Par parameter
function [Kw, K_theta,C_theta] = fcn(Par)

% Calculating Pitching stiffness
Kw_fl = Par.Ks_f.*(Par.Motion_ratio_f)^2; 
Kw_fr = Par.Ks_f.*(Par.Motion_ratio_f)^2;
Kw_rl = Par.Ks_r.*(Par.Motion_ratio_r)^2;
Kw_rr = Par.Ks_r.*(Par.Motion_ratio_r)^2;

K_theta = (Kw_fl + Kw_fr).*(Par.Lf)^2 + (Kw_rl + Kw_rr).*(Par.Lr)^2;

% Calculating Pitch Damping
Cw_fl = Par.C_damp_f.*(Par.Motion_ratio_f)^2;
Cw_fr = Par.C_damp_f.*(Par.Motion_ratio_f)^2;
Cw_rl = Par.C_damp_r.*(Par.Motion_ratio_r)^2;
Cw_rr = Par.C_damp_r.*(Par.Motion_ratio_r)^2;

C_theta = (Cw_fl + Cw_fr).*(Par.Lf)^2 + (Cw_rl + Cw_rr).*(Par.Lr)^2;

Kw = [Kw_fl;Kw_fr;Kw_rl;Kw_rr];

== matlab function e_Aerodynamics_added/roll and pitch angles/Phi_constants ==
  data: K_phi output; C_phi output; Par parameter
function [K_phi,C_phi] = fcn(Par)

% Calculating Pitching stiffness
Kw_fl = Par.Ks_f.*(Par.Motion_ratio_f)^2; 
Kw_fr = Par.Ks_f.*(Par.Motion_ratio_f)^2;
Kw_rl = Par.Ks_r.*(Par.Motion_ratio_r)^2;
Kw_rr = Par.Ks_r.*(Par.Motion_ratio_r)^2;

K_phi = (Kw_fl + Kw_fr).*(Par.TW/2)^2 + (Kw_rl + Kw_rr).*(Par.TW/2)^2;

% Calculating Pitch Damping
Cw_fl = Par.C_damp_f.*(Par.Motion_ratio_f)^2;
Cw_fr = Par.C_damp_f.*(Par.Motion_ratio_f)^2;
Cw_rl = Par.C_damp_r.*(Par.Motion_ratio_r)^2;
Cw_rr = Par.C_damp_r.*(Par.Motion_ratio_r)^2;

C_phi = (Cw_fl + Cw_fr).*(Par.TW/2)^2 + (Cw_rl + Cw_rr).*(Par.TW/2)^2;

== matlab function e_Aerodynamics_added/Normal Loads ==
  data: Fz_New output; phi input; theta input; Kw input; Vel input; Par parameter; Fs output size=4; Farb output; F_aero_total output
function [Fz_New,Fs,Farb,F_aero_total] = fcn(phi,theta,Kw,Vel,Par)
    %#codegen
    % Inputs:
    %   ax_g, ay_g : Acceleration 
    %   m          : Mass [kg]
    %   Par        : Structure with field .g, .WB, .TW, .CG_h, .WD_R, .K_roll_F

    % 1. Constants
    g = Par.g;
    L = Par.WB;     % Wheelbase
    T = Par.TW;     % Track Width
    h = Par.CG_h;   % CG Height
    m = Par.m;
   
    % Front and rear Wheelbase
    Lf = L*0.51;
    Lr = L*0.49;

    % Static load 
    F_static = m*g;
    
    % Vertical deflection of each suspension
    zsfl = Lf*theta + (T/2)*phi;
    zsfr = Lf*theta - (T/2)*phi;
    zsrl = -Lr*theta + (T/2)*phi;
    zsrr = -Lr*theta - (T/2)*phi;

    % Spring force at each wheel
    Fs_fl = Kw(1)*zsfl;
    Fs_fr = Kw(2)*zsfr;
    Fs_rl = Kw(3)*zsrl;
    Fs_rr = Kw(4)*zsrr;

    % Calculation of Anti roll bar forces at each wheel
    delta_zf = zsfl - zsfr;
    delta_zr = zsrl - zsrr;

    F_arb_fl = Par.K_arb_f*delta_zf/2;
    F_arb_fr = -Par.K_arb_f*delta_zf/2;
    F_arb_rl = Par.K_arb_r*delta_zr/2;
    F_arb_rr = -Par.K_arb_r*delta_zr/2;

    % Net normal force on each wheel
    F_static_per_wheel = F_static/4;

    Fz_FL = F_static_per_wheel - Fs_fl - F_arb_fl;
    Fz_FR = F_static_per_wheel - Fs_fr - F_arb_fr;
    Fz_RL = F_static_per_wheel - Fs_rl - F_arb_rl;
    Fz_RR = F_static_per_wheel - Fs_rr - F_arb_rr;
   
    % Safety Clamp (Wheelie prevention)
    Min_Load = 10; 

    Fz_FL = max(Fz_FL, Min_Load);
    Fz_FR = max(Fz_FR, Min_Load);
    Fz_RL = max(Fz_RL, Min_Load);
    Fz_RR = max(Fz_RR, Min_Load);

    % Fz_out = [Fz_FL; Fz_FR; Fz_RL; Fz_RR];
    
    Fs = [Fs_fl;Fs_fr;Fs_rl;Fs_rr];
    Farb = [F_arb_fl;F_arb_fr;F_arb_rl;F_arb_rr];
   
% F_aero = 0.5 * rho * Cl * A * v^2
   F_aero_total = -0.5 * 1.225 * Par.Cl * Par.Area * Vel^2;

% Distribute Aero (Usually based on Center of Pressure, CP)
  
   aero_Fz_FL = Fz_FL + 0.5 * F_aero_total * (1 - Par.CP_Rear);
   aero_Fz_FR = Fz_FR + 0.5 * F_aero_total * (1 - Par.CP_Rear);
   aero_Fz_RL = Fz_RL + 0.5*F_aero_total*(Par.CP_Rear);
   aero_Fz_RR = Fz_RR + 0.5*F_aero_total*(Par.CP_Rear);

   Fz_new = [aero_Fz_FL;aero_Fz_FR;aero_Fz_RL;aero_Fz_RR];
   Fz_New = Fz_new;
   
end

== matlab function e_Aerodynamics_added/Simplified Tire Model ==
  data: Fz input; Fx output size=4; slip_ratios input; slip_angles input; camber_angles input; Fy output size=4; Mz output size=4; Mu_x output size=4; Mu_y output size=4; TireData parameter; Par parameter
function [Fx, Fy, Mz, Mu_x, Mu_y] = fcn(Fz, slip_ratios, slip_angles, camber_angles, TireData,Par)
%#codegen
% =========================================================================
%  VECTORIZED MAGIC FORMULA 5.2 (4-WHEEL)
%  Computes tire physics for all 4 corners simultaneously using element-wise math.
%
%  INPUTS (All 4x1 Vectors):
%    Fz    : Vertical Loads [N] -> [FL; FR; RL; RR]
%    Kappa : Slip Ratios [-]
%    Alpha : Slip Angles [rad]
%    Gamma : Camber Angles [rad]
%    TireData : Parameter Struct (Must be loaded in Base Workspace)
%
%  OUTPUTS (All 4x1 Vectors):
%    Fx    : Longitudinal Force [N]
%    Fy    : Lateral Force [N]
%    Mz    : Self-Aligning Torque [Nm]
%    Mu_x  : Long. Friction Coeff [-]
%    Mu_y  : Lat. Friction Coeff [-]
% =========================================================================

    % 1. EXTRACT PARAMETERS (Scalars)
    p = TireData;
    s = TireData.Scales;
    Fz0 = p.Fz0;
    R0  = p.R0;
    par = Par;
    % 2. INPUT SAFETY & NORMALIZATION
    % Clamp negative loads to 0 (Tires can't pull ground)
    Fz_safe = max(Fz, 0); 
    
    % Avoid division by zero for Mu calculations later
    Fz_denom = max(Fz_safe, 1.0); 

    % Normalized Load (dfz) - Vectorized
    dfz = (Fz_safe - Fz0) ./ Fz0;

    % ---------------------------------------------------------------------
    % A. LONGITUDINAL FORCE (Fx) - VECTORIZED
    % ---------------------------------------------------------------------
    Cx = p.PCX1 * s.LCX;
    
    % Friction Coeff Mu_x
    mu_x_base = (p.PDX1 + p.PDX2 .* dfz) .* (1 - p.PDX3 .* camber_angles.^2) .* s.LMUX;
    Dx = mu_x_base .* Fz_safe;
    
    % Stiffness Kx
    Kx = Fz_safe .* (p.PKX1 + p.PKX2 .* dfz) .* exp(p.PKX3 .* dfz) .* s.LKX;
    
    % Stiffness Factor Bx
    Bx = Kx ./ (Cx .* Dx + 1e-6); 
    
    % Shifts (Horizontal & Vertical)
    Shx = (p.PHX1 + p.PHX2 .* dfz) .* s.LHX;
    Svx = Fz_safe .* (p.PVX1 + p.PVX2 .* dfz) .* s.LVX;
    
    % Composite Slip
    k_s = slip_ratios + Shx;
    
    % Curvature Ex (Sign Dependent)
    Ex = (p.PEX1 + p.PEX2 .* dfz + p.PEX3 .* dfz.^2) .* (1 - p.PEX4 .* sign(k_s)) .* s.LEX;
    Ex(Ex > 1) = 1; % Clamp
    
    % Calculation
    Bx_k = Bx .* k_s;
    Fx = Dx .* sin(Cx .* atan(Bx_k - Ex .* (Bx_k - atan(Bx_k)))) + Svx;

    % ---------------------------------------------------------------------
    % B. LATERAL FORCE (Fy) - VECTORIZED
    % ---------------------------------------------------------------------
    Cy = p.PCY1 * s.LCY;
    
    % Friction Coeff Mu_y
    mu_y_base = (p.PDY1 + p.PDY2 .* dfz) .* (1 - p.PDY3 .* camber_angles.^2) .* s.LMUY;
    Dy = mu_y_base .* Fz_safe;
    
    % Cornering Stiffness Ky (Trig Form)
    Ky = p.PKY1 .* Fz0 .* sin(2 .* atan(Fz_safe ./ (p.PKY2 .* Fz0))) .* (1 - p.PKY3 .* abs(camber_angles)) .* s.LKY;
    
    % Poly fallback check (if PKY2 implies poly form)
    if (Ky(1) < 1)
        Ky = Fz_safe .* (p.PKY1 + p.PKY2 .* dfz) .* s.LKY;
    end
    
    By = Ky ./ (Cy .* Dy + 1e-6);
    
    % Shifts
    Shy = (p.PHY1 + p.PHY2 .* dfz) .* s.LHY;
    Svy = Fz_safe .* (p.PVY1 + p.PVY2 .* dfz) .* s.LVY;
    
    a_s = slip_angles + 0*Shy;
    
    % Curvature Ey (Sign Dependent)
    Ey = (p.PEY1 + p.PEY2 .* dfz) .* (1 - (p.PEY3 + p.PEY4 .* camber_angles) .* sign(a_s)) .* s.LEY;
    Ey(Ey > 1) = 1;
    
    % Calculation
    By_a = By .* a_s;
    Fy = -(Dy .* sin(Cy .* atan(By_a - Ey .* (By_a - atan(By_a)))) + 0*Svy);

    % ---------------------------------------------------------------------
    % C. SELF-ALIGNING TORQUE (Mz) - VECTORIZED
    % ---------------------------------------------------------------------
    % Peak Trail Dt
    Dt = (p.QDZ1 + p.QDZ2 .* dfz) .* (1 - p.QDZ3 .* abs(camber_angles)) .* R0 .* s.LTR;
    
    % Trail Slope Bt
    Bt = (p.QBZ1 + p.QBZ2 .* dfz + p.QBZ3 .* dfz.^2) .* (1 + p.QBZ4 .* abs(camber_angles)) .* (s.LKY / s.LMUY);
    
    Ct = p.QCZ1; % Scalar
    Et = (p.QEZ1 + p.QEZ2 .* dfz + p.QEZ3 .* dfz.^2);
    
    % Trail 't' Calculation(Pneumatic trail)
    Bt_a = Bt .* a_s;
    alpha_t = Bt_a - Et .* (Bt_a - atan(Bt_a));
    t = Dt .* cos(Ct .* atan(alpha_t)) .* cos(a_s);

    % Trail 'tm' Calculation(mechanical trail)
    tm = par.R0.*tan(par.Caster_static);

    % Residual Mzr
    Dr = Fz_safe .* R0 .* (p.QDZ6 + p.QDZ7 .* dfz) .* s.LRES;
    Br = 10;
    Mzr = Dr .* cos(atan(Br .* a_s));
    
    % Final Mz (Standard Restoring: Negative Slope)
    % Note: If you want positive slope (sharp tune from before), multiply term by -1.
    Mz = -(t+tm).*Fy + Mzr;

    % ---------------------------------------------------------------------
    % D. OUTPUTS (Zero out lifted wheels)
    % ---------------------------------------------------------------------
    % Friction Coeffs
    Mu_x = Fx ./ Fz_denom;
    Mu_y = Fy ./ Fz_denom;

    % Clean up lifted wheels (Fz <= 0)
    % lifted_idx = Fz <= 0;
    % Fx(lifted_idx) = 0;
    % Fy(lifted_idx) = 0;
    % Mz(lifted_idx) = 0;
    % Mu_x(lifted_idx) = 0;
    % Mu_y(lifted_idx) = 0;

end

== matlab function e_Aerodynamics_added/slip ratios ==
  data: Vx input; Vy input; slip_ratios output; yawrate input; Omega input; Steer_FL input; Steer_FR input; Par parameter
function slip_ratios = fcn(Vx,Vy, yawrate, Omega,Steer_FL,Steer_FR, Par)
%#codegen


    % 1. Constants
    T = Par.TW;
    Re = Par.R0;
    half_T = T / 2;
    a= Par.a;
    b=Par.b;
    r = yawrate;
    % 2 Yaw Rate Correction (Kinematics)
    
    Vx_FL = Vx - yawrate * half_T;  % Left
    Vx_FR = Vx + yawrate * half_T;  % Right
    Vx_RL = Vx - yawrate * half_T;
    Vx_RR = Vx + yawrate * half_T;
    
    Vx_vec = [Vx_FL; Vx_FR; Vx_RL; Vx_RR];
    
    Vy_FL = Vy + r * a;
    Vy_FR = Vy+ r * a;
    Vy_RL = Vy- r * b;
    Vy_RR = Vy- r * b;

    Vy_vec = [Vy_FL; Vy_FR; Vy_RL; Vy_RR];
    Delta = [Steer_FL;Steer_FR;0;0];
    % 3. Slip Angle Correction (Projection)
 
    V_road_plane = Vx_vec .* cos(Delta) + Vy_vec .* sin(Delta);

    % 4. Calculate Wheel Linear Speed
    V_wheel = Omega .* Re;

    % 5. Calculate Slip Ratio
    V_safe_threshold = 0.1; 
    V_ref = max(abs(V_road_plane), V_safe_threshold);
    
    slip_ratios_raw = (V_wheel - V_road_plane) ./ V_ref;
    slip_ratios = min(max(slip_ratios_raw,-1),1);
end
